simulink model "mwave_remover"  (R2014a)
settings: Solver=ode45  StartTime=0.0  StopTime=10.0  RelTol=1e-3
libraries: dspmtrx3 x2, dspinverses x1
settings Model: Creator=BETHEL.OSUAGWU  LastModifiedBy=BETHEL.OSUAGWU

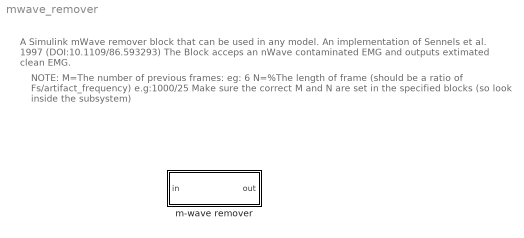
== system mwave_remover ==
  note: NOTE:
      | M=The number of previous frames: eg: 6
      | N=%The length of frame (should be a ratio of Fs/artifact_frequency) e.g:1000/25
      | Make sure the correct M and N are set in the specified blocks (so look inside the subsystem)
  note: A Simulink mWave remover block that can be used in any model. An implementation of Sennels et al. 1997 (DOI:10.1109/86.593293)
      | The Block acceps an nWave contaminated EMG and outputs extimated clean EMG.
  m-wave remover : Subsystem

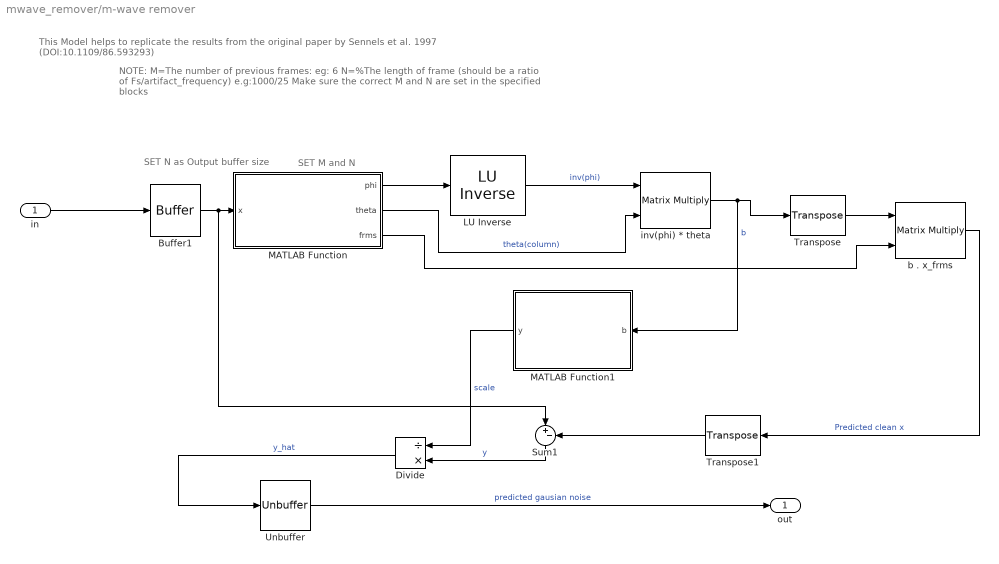
== system mwave_remover/m-wave remover ==
  note: NOTE:
      | M=The number of previous frames: eg: 6
      | N=%The length of frame (should be a ratio of Fs/artifact_frequency) e.g:1000/25
      | Make sure the correct M and N are set in the specified blocks
  note: SET N as Output
      | buffer size
  note: SET M and N
  note: This Model helps to replicate the results from the original paper by Sennels et al. 1997 (DOI:10.1109/86.593293)
  in : Inport
  " LU Inverse" : dspinverses/ LU Inverse
  Buffer1 : Buffer  N=40  TreatMby1Signals=One channel
  Divide : Product  Inputs=/*
  MATLAB Function : MATLAB Function  TreatAsAtomicUnit=on
  MATLAB Function1 : MATLAB Function  TreatAsAtomicUnit=on
  Sum1 : Sum  Inputs=|+-
  Transpose : dspmtrx3/Transpose  Hermitian=off  overflowFlag=off
  Transpose1 : dspmtrx3/Transpose  Hermitian=off  overflowFlag=off
  Unbuffer : Unbuffer  SampleBasedProcessing=Same as frame based
  b . x_frms : Product  Multiplication=Matrix(*)
  inv(phi) * theta : Product  Multiplication=Matrix(*)
  out : Outport
  wires:
  Buffer1/1 -> Sum1/1, MATLAB Function/1(x)
  MATLAB Function/1(phi) -> " LU Inverse"/1
  MATLAB Function/2(theta) -> inv(phi) * theta/2  "theta(column)"
  " LU Inverse"/1 -> inv(phi) * theta/1  "inv(phi)"
  inv(phi) * theta/1 -> MATLAB Function1/1(b), Transpose/1  "b"
  Unbuffer/1 -> out/1  "predicted gausian noise"
  MATLAB Function/3(frms) -> b . x_frms/2
  Transpose/1 -> b . x_frms/1
  b . x_frms/1 -> Transpose1/1  "Predicted clean x"
  Transpose1/1 -> Sum1/2
  Sum1/1 -> Divide/2  "y"
  MATLAB Function1/1(y) -> Divide/1  "scale"
  Divide/1 -> Unbuffer/1  "y_hat"
  in/1 -> Buffer1/1

== matlab function mwave_remover/m-wave remover/MATLAB Function ==
  data: x input; phi output double; theta output; frms output
function [phi,theta,frms] = fcn(x)
%#codegen
persistent t_sample phi_mem  frms_mem ;

%General param
M=6; %The number of previous frames 
N=40; %The length of frame (should be a ratio of Fs/artifact_frequency)

% Performance parameter
freshPhi =1;% when =1:recompute phi(covariance matix) all the phi; when =0:update phi with only new values

if isempty(t_sample)
    t_sample=0;
    frms_mem=zeros(M,N);
    
    phi_mem=zeros(M,M);
end
t_sample=t_sample+1;

%make x a row vector
x=x';


%% compute phi
frms=frms_mem;
%equ 7 and 8
if(freshPhi)
    % compute phi fresh all the time
    phi=(frms*frms');
else
    %we can compute only the required column (first) and row (first)of phi
    %matrix and push the new values into phi
    phi_mem(2:end,2:end)=phi_mem(1:end-1,1:end-1);
    phi_mem(1,:)=frms(1,:)*frms';
    phi_mem(:,1)=phi_mem(1,:)';
    %phi-phi_mem
    phi=phi_mem;
end


%% compute theta
theta=(x*frms')';
%t_sample
%if t_sample==15
%    y=4;
%end


%% update frame
frms_mem(2:end,:)=frms_mem(1:end-1,:);
frms_mem(1,:)=x;

== matlab function mwave_remover/m-wave remover/MATLAB Function1 ==
  data: b input; y output
function y = fcn(b)
%#codegen


y = sqrt(1+sum(b.^2));
%       OR
%y = (1+sum(b));%approximated for speed
